simulink model "model1"  (R2025b)
settings: Solver=VariableStepAuto  StartTime=0.0  StopTime=10.0  RelTol=1e-3
settings Model: Creator=FAY1GA  LastModifiedBy=FAY1GA

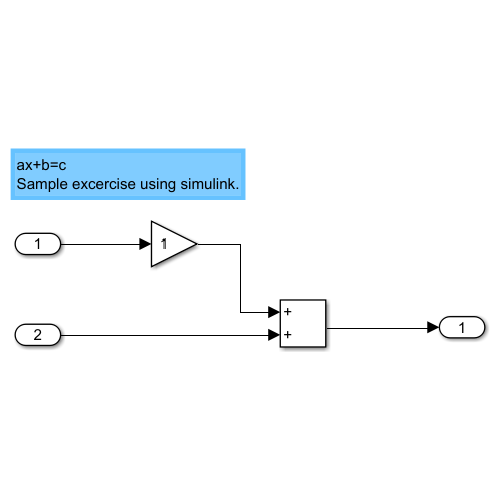
[thumbnail: Simulink's stored preview of the top-level diagram]
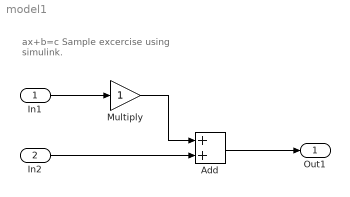
== system model1 ==
  note: ax+b=c
      | Sample excercise using simulink.
  In1 : Inport
  In2 : Inport  Port=2
  Add : Sum
  Multiply : Gain
  Out1 : Outport
  wires:
  In1/1 -> Multiply/1
  Multiply/1 -> Add/1
  In2/1 -> Add/2
  Add/1 -> Out1/1
